simulink library "InputBlocks_library"  (R2018b)
settings: Solver=VariableStepAuto  StartTime=0.0  StopTime=10.0  RelTol=1e-3
undefined symbols (not defined in the file): aircraft, trimPoint
libraries: unit_conversions_lib x5, se2a_command_lib x2
settings Model: ModifiedByFormat=dcava  Creator=cava_da  LastModifiedBy=dcava

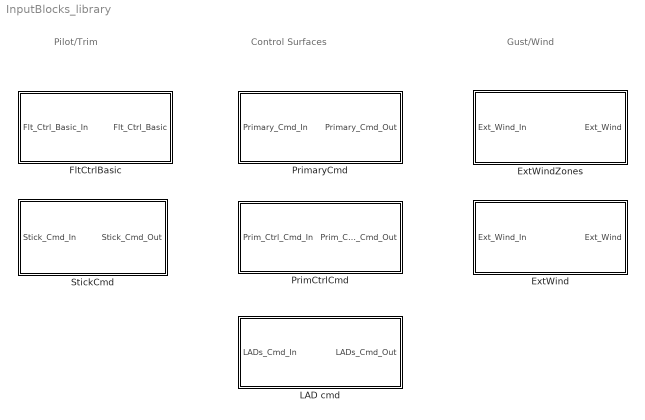
== system InputBlocks_library ==
  note: Gust/Wind
  note: Control Surfaces
  note: Pilot/Trim
  ExtWind : Subsystem
  ExtWindZones : Subsystem
  FltCtrlBasic : Subsystem  mask{n_ail_pair=aircraft.wing_main.params.num_flaps/2, n_LADs=aircraft.wing_main.params.num_lads, actuators=aircraft.actuators}
      mask prompts: n_ail_pair "Number of aileron pairs:"; n_LADs "Number of LADs:"; actuators "Actuator parameter struct:"
  LAD cmd : Subsystem  mask{num_lads=1}
      mask prompts: num_lads "Number of LADs"
      mask DialogControl DescGroupVar Prompt: Load alleviation devices commands
  PrimCtrlCmd : Subsystem  mask{n_ail_pairs=aircraft.wing_main.params.num_flaps/2, n_LADs=aircraft.wing_main.params.num_lads, actuators=aircraft.actuators}
      mask prompts: n_ail_pairs "Number of aileron pairs:"; n_LADs "Number of LADs:"; actuators "Actuator parameter struct:"
  PrimaryCmd : Subsystem
  StickCmd : Subsystem

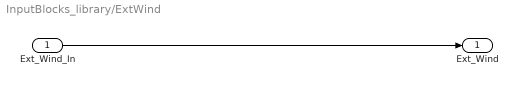
== system InputBlocks_library/ExtWind ==
  Ext_Wind_In : Inport
  Ext_Wind : Outport  VectorParamsAs1DForOutWhenUnconnected=off
  wires:
  Ext_Wind_In/1 -> Ext_Wind/1

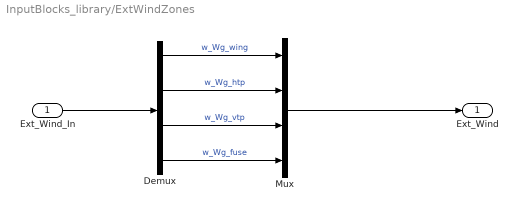
== system InputBlocks_library/ExtWindZones ==
  Ext_Wind_In : Inport
  Demux : Demux
  Mux : Mux
  Ext_Wind : Outport  VectorParamsAs1DForOutWhenUnconnected=off
  wires:
  Ext_Wind_In/1 -> Demux/1
  Demux/1 -> Mux/1  "w_Wg_wing"
  Demux/2 -> Mux/2  "w_Wg_htp"
  Demux/3 -> Mux/3  "w_Wg_vtp"
  Demux/4 -> Mux/4  "w_Wg_fuse"
  Mux/1 -> Ext_Wind/1

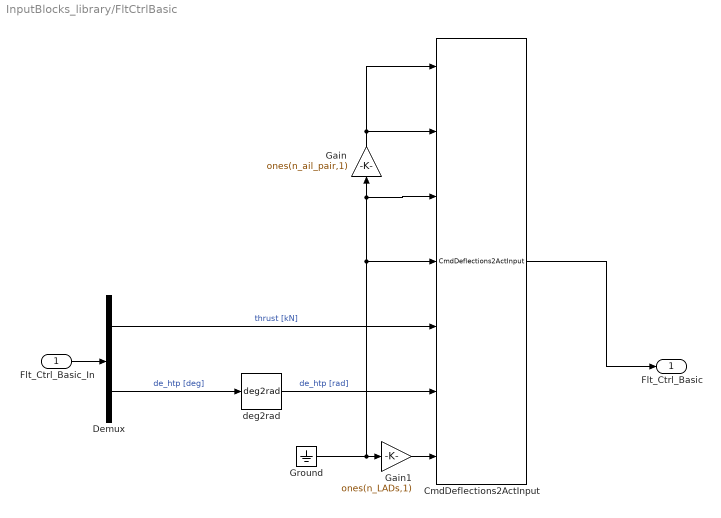
== system InputBlocks_library/FltCtrlBasic ==
  Flt_Ctrl_Basic_In : Inport
  CmdDeflections2ActInput : se2a_command_lib/CmdDeflections2ActInput  actuators=actuators
      settings: SourceProductName=SE2A library
  Demux : Demux  Outputs=2
  Gain : Gain  Gain=ones(n_ail_pair,1)
  Gain1 : Gain  Gain=ones(n_LADs,1)
  Ground : Ground
  deg2rad : unit_conversions_lib/deg2rad
      settings: SourceProductName=LADAC
  Flt_Ctrl_Basic : Outport  VectorParamsAs1DForOutWhenUnconnected=off
  wires:
  Gain1/1 -> CmdDeflections2ActInput/7
  Gain/1 -> CmdDeflections2ActInput/1, CmdDeflections2ActInput/2
  CmdDeflections2ActInput/1 -> Flt_Ctrl_Basic/1
  Ground/1 -> Gain/1, CmdDeflections2ActInput/3, CmdDeflections2ActInput/4, Gain1/1
  deg2rad/1 -> CmdDeflections2ActInput/6  "de_htp [rad]"
  Demux/2 -> deg2rad/1  "de_htp [deg]"
  Demux/1 -> CmdDeflections2ActInput/5  "thrust [kN]"
  Flt_Ctrl_Basic_In/1 -> Demux/1

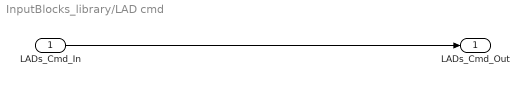
== system InputBlocks_library/LAD cmd ==
  LADs_Cmd_In : Inport  PortDimensions=num_lads
  LADs_Cmd_Out : Outport  VectorParamsAs1DForOutWhenUnconnected=off
  wires:
  LADs_Cmd_In/1 -> LADs_Cmd_Out/1

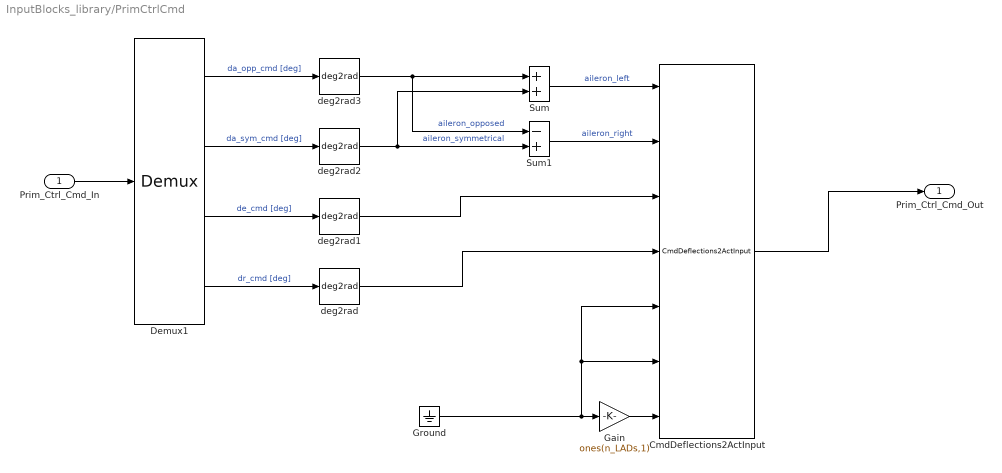
== system InputBlocks_library/PrimCtrlCmd ==
  Prim_Ctrl_Cmd_In : Inport
  CmdDeflections2ActInput : se2a_command_lib/CmdDeflections2ActInput  actuators=actuators
      settings: SourceProductName=SE2A library
  Demux1 : Demux  Outputs=[n_ail_pairs, n_ail_pairs, 1, 1]
      settings: DisplayOption=none
  Gain : Gain  Gain=ones(n_LADs,1)
  Ground : Ground
  Sum : Sum
  Sum1 : Sum  Inputs=-+
  deg2rad{,1..3} (4 alike) : unit_conversions_lib/deg2rad
      settings: SourceProductName=LADAC
  Prim_Ctrl_Cmd_Out : Outport  VectorParamsAs1DForOutWhenUnconnected=off
  wires:
  Gain/1 -> CmdDeflections2ActInput/7
  CmdDeflections2ActInput/1 -> Prim_Ctrl_Cmd_Out/1
  Ground/1 -> CmdDeflections2ActInput/6, CmdDeflections2ActInput/5, Gain/1
  deg2rad/1 -> CmdDeflections2ActInput/4
  Sum1/1 -> CmdDeflections2ActInput/2  "aileron_right"
  Sum/1 -> CmdDeflections2ActInput/1  "aileron_left"
  deg2rad2/1 -> Sum1/2, Sum/2  "aileron_symmetrical"
  deg2rad3/1 -> Sum1/1, Sum/1  "aileron_opposed"
  Prim_Ctrl_Cmd_In/1 -> Demux1/1
  Demux1/1 -> deg2rad3/1  "da_opp_cmd [deg]"
  Demux1/4 -> deg2rad/1  "dr_cmd [deg]"
  Demux1/3 -> deg2rad1/1  "de_cmd [deg]"
  Demux1/2 -> deg2rad2/1  "da_sym_cmd [deg]"
  deg2rad1/1 -> CmdDeflections2ActInput/3

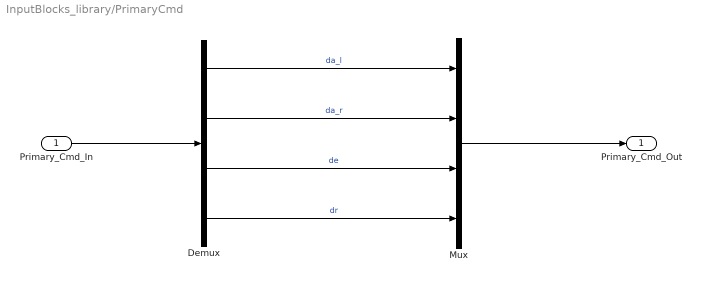
== system InputBlocks_library/PrimaryCmd ==
  Primary_Cmd_In : Inport
  Demux : Demux
  Mux : Mux
  Primary_Cmd_Out : Outport  VectorParamsAs1DForOutWhenUnconnected=off
  wires:
  Primary_Cmd_In/1 -> Demux/1
  Mux/1 -> Primary_Cmd_Out/1
  Demux/1 -> Mux/1  "da_l"
  Demux/4 -> Mux/4  "dr"
  Demux/3 -> Mux/3  "de"
  Demux/2 -> Mux/2  "da_r"

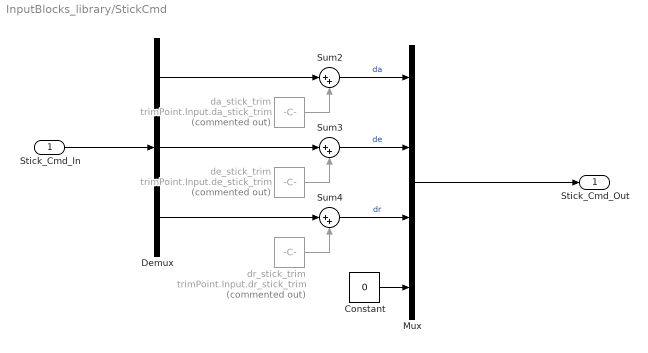
== system InputBlocks_library/StickCmd ==
  Stick_Cmd_In : Inport
  Constant : Constant  Value=0
  Demux : Demux  Outputs=3
  Mux : Mux
  Sum2 : Sum  Inputs=|++
  Sum3 : Sum  Inputs=|++
  Sum4 : Sum  Inputs=|++
  da_stick_trim : Constant  Commented=on  Value=trimPoint.Input.da_stick_trim
  de_stick_trim : Constant  Commented=on  Value=trimPoint.Input.de_stick_trim
  dr_stick_trim : Constant  Commented=on  Value=trimPoint.Input.dr_stick_trim
  Stick_Cmd_Out : Outport  VectorParamsAs1DForOutWhenUnconnected=off
  wires:
  Demux/1 -> Sum2/1
  Constant/1 -> Mux/4
  Sum3/1 -> Mux/2  "de"
  dr_stick_trim/1 -> Sum4/2
  de_stick_trim/1 -> Sum3/2
  Demux/3 -> Sum4/1
  Sum4/1 -> Mux/3  "dr"
  Sum2/1 -> Mux/1  "da"
  da_stick_trim/1 -> Sum2/2
  Demux/2 -> Sum3/1
  Mux/1 -> Stick_Cmd_Out/1
  Stick_Cmd_In/1 -> Demux/1
